simulink model "holiday6"  (R2019a)
settings: Solver=VariableStepAuto  StartTime=0.0  StopTime=10.0  RelTol=1e-3
libraries: simulink x1
settings Model: Creator=Aditya  LastModifiedBy=Aditya

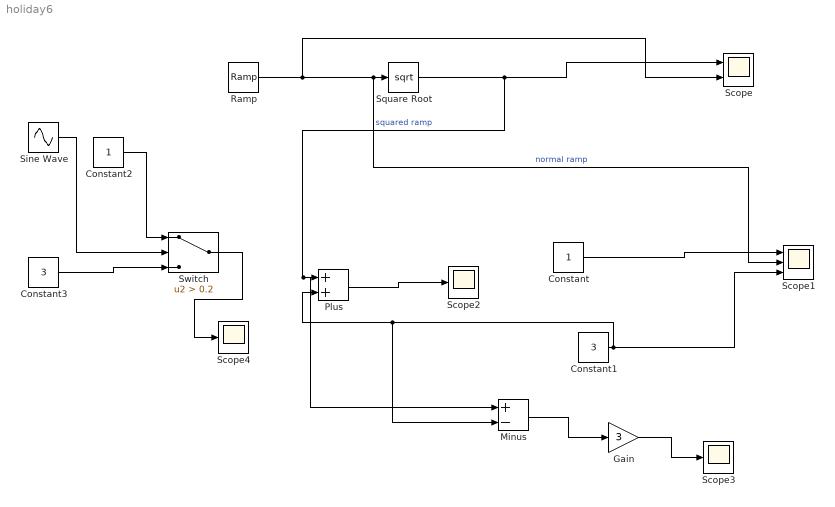
== system holiday6 ==
  Constant : Constant
  Constant1 : Constant  Value=3
  Constant2 : Constant
  Constant3 : Constant  Value=3
  Gain : Gain  Gain=3
  Minus : Sum  Inputs=+-
  Plus : Sum
  Ramp : simulink/Sources/Ramp  slope=3  start=0  InitialOutput=0
  Scope : Scope  NumInputPorts=2
  Scope1 : Scope  NumInputPorts=3
  Scope2 : Scope
  Scope3 : Scope
  Scope4 : Scope
  Sine Wave : Sin  Amplitude=5  SampleTime=0
  Square Root : Sqrt  SaturateOnIntegerOverflow=on
  Switch : Switch  Criteria=u2 > Threshold  Threshold=0.2
  wires:
  Ramp/1 -> Scope/2, Scope1/2, Square Root/1  "normal ramp"
  Square Root/1 -> Minus/1, Plus/1, Scope/1  "squared ramp"
  Constant/1 -> Scope1/1
  Constant1/1 -> Minus/2, Plus/2, Scope1/3
  Plus/1 -> Scope2/1
  Minus/1 -> Gain/1
  Gain/1 -> Scope3/1
  Constant2/1 -> Switch/1
  Constant3/1 -> Switch/3
  Sine Wave/1 -> Switch/2
  Switch/1 -> Scope4/1
